simulink model "DynamicModel_Unicycle"  (R2018a)
settings: Solver=ode4  StartTime=0.0  StopTime=10  FixedStep=0.01  RelTol=1e-3
settings Model: Creator=Yuri  LastModifiedBy=Yuri

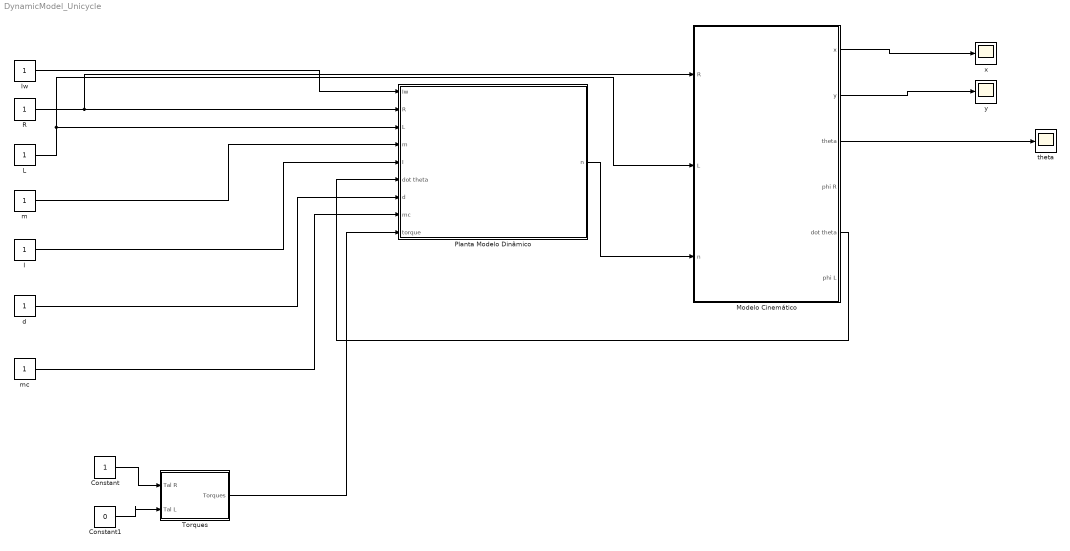
== system DynamicModel_Unicycle ==
  Constant : Constant
  Constant1 : Constant  Value=0
  I : Constant
  Iw : Constant
  L : Constant
  Modelo Cinemático : Subsystem
  Planta Modelo Dinâmico : Subsystem
  R : Constant
  Torques : Subsystem
  d : Constant
  m : Constant
  mc : Constant
  "theta " : Scope
  x : Scope
  y : Scope
  wires:
  R/1 -> Modelo Cinemático/1(R), Planta Modelo Dinâmico/2(R)
  L/1 -> Modelo Cinemático/2(L), Planta Modelo Dinâmico/3(L)
  Iw/1 -> Planta Modelo Dinâmico/1(Iw)
  m/1 -> Planta Modelo Dinâmico/4(m)
  I/1 -> Planta Modelo Dinâmico/5(I)
  d/1 -> Planta Modelo Dinâmico/7(d)
  mc/1 -> Planta Modelo Dinâmico/8(mc)
  Torques/1("Torques ") -> Planta Modelo Dinâmico/9(torque)
  Constant/1 -> Torques/1(Tal R)
  Constant1/1 -> Torques/2(Tal L)
  Modelo Cinemático/3(theta) -> "theta "/1
  Planta Modelo Dinâmico/1(n) -> Modelo Cinemático/3(n)
  Modelo Cinemático/1(x) -> x/1
  Modelo Cinemático/2(y) -> y/1
  Modelo Cinemático/5(dot theta) -> Planta Modelo Dinâmico/6(dot theta)

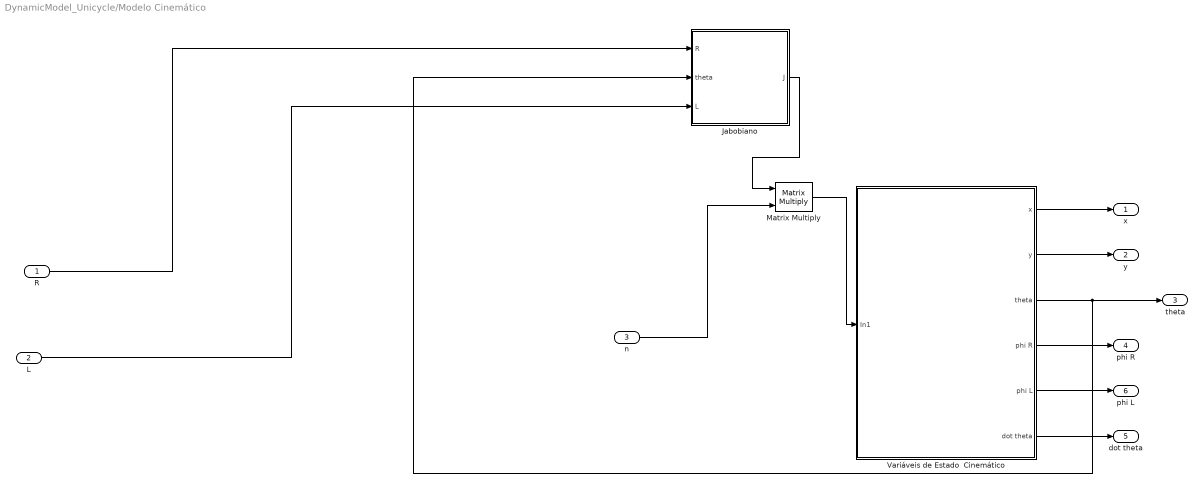
== system DynamicModel_Unicycle/Modelo Cinemático ==
  R : Inport
  L : Inport  Port=2
  n : Inport  Port=3
  "Jabobiano " : Subsystem
  Matrix Multiply : Product  Multiplication=Matrix(*)
  Variáveis de Estado  Cinemático : Subsystem
  x : Outport
  y : Outport  Port=2
  theta : Outport  Port=3
  phi R : Outport  Port=4
  dot theta : Outport  Port=5
  phi L : Outport  Port=6
  wires:
  Matrix Multiply/1 -> Variáveis de Estado  Cinemático/1(In1)
  "Jabobiano "/1(J) -> Matrix Multiply/1
  Variáveis de Estado  Cinemático/5(phi L) -> phi L/1
  Variáveis de Estado  Cinemático/1(x) -> x/1
  Variáveis de Estado  Cinemático/3(theta) -> theta/1, "Jabobiano "/2(theta)
  Variáveis de Estado  Cinemático/6(dot theta) -> dot theta/1
  R/1 -> "Jabobiano "/1(R)
  Variáveis de Estado  Cinemático/4(phi R) -> phi R/1
  Variáveis de Estado  Cinemático/2(y) -> y/1
  L/1 -> "Jabobiano "/3(L)
  n/1 -> Matrix Multiply/2

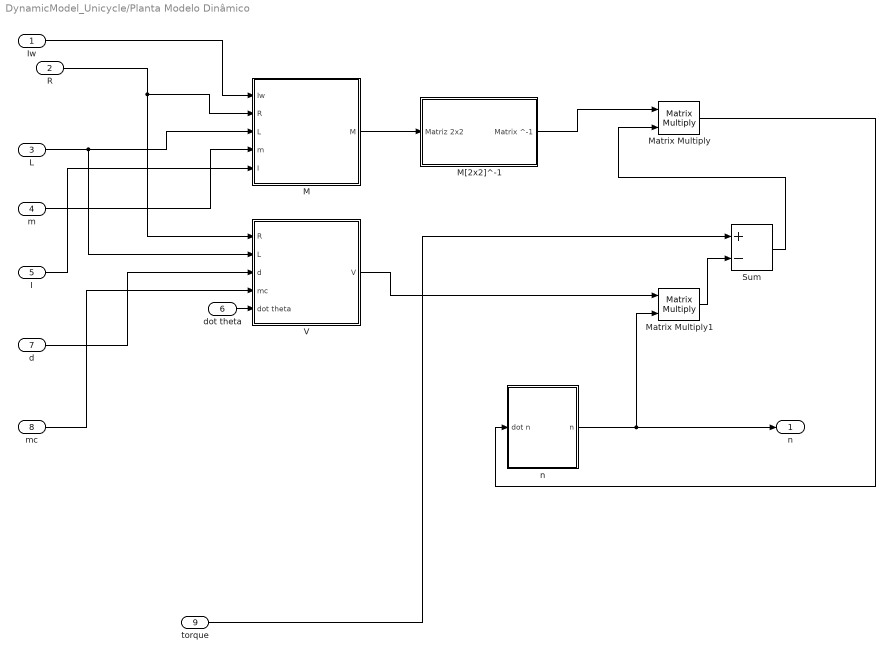
== system DynamicModel_Unicycle/Planta Modelo Dinâmico ==
  Iw : Inport
  R : Inport  Port=2
  L : Inport  Port=3
  m : Inport  Port=4
  I : Inport  Port=5
  dot theta : Inport  Port=6
  d : Inport  Port=7
  mc : Inport  Port=8
  torque : Inport  Port=9
  " n" : Subsystem
  M : Subsystem
  M[2x2]^-1 : Subsystem
  Matrix Multiply : Product  Multiplication=Matrix(*)
  Matrix Multiply1 : Product  Multiplication=Matrix(*)
  Sum : Sum  Inputs=+-
  V : Subsystem
  n : Outport
  wires:
  Matrix Multiply1/1 -> Sum/2
  Sum/1 -> Matrix Multiply/2
  " n"/1("n ") -> n/1, Matrix Multiply1/2
  M[2x2]^-1/1(Matrix ^-1) -> Matrix Multiply/1
  Matrix Multiply/1 -> " n"/1(dot n)
  torque/1 -> Sum/1
  L/1 -> V/2(L), M/3(L)
  mc/1 -> V/4(mc)
  R/1 -> M/2(R), V/1(R)
  dot theta/1 -> V/5(dot theta)
  Iw/1 -> M/1(Iw)
  I/1 -> M/5(I)
  m/1 -> M/4(m)
  d/1 -> V/3(d)
  M/1(M) -> M[2x2]^-1/1("Matriz 2x2 ")
  V/1(V) -> Matrix Multiply1/1

== system DynamicModel_Unicycle/Torques ==
  Tal R : Inport
  Tal L : Inport  Port=2
  Mux : Mux  Inputs=2
  "[2,1]" : Reshape  OutputDimensionality=Customize  OutputDimensions=[2,1]
  "Torques " : Outport
  wires:
  Tal R/1 -> Mux/1
  Tal L/1 -> Mux/2
  Mux/1 -> "[2,1]"/1
  "[2,1]"/1 -> "Torques "/1

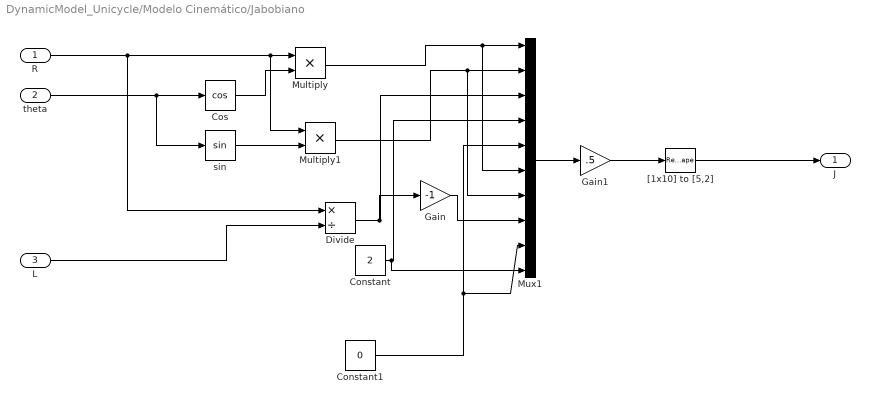
== system DynamicModel_Unicycle/Modelo Cinemático/Jabobiano  ==
  R : Inport
  theta : Inport  Port=2
  L : Inport  Port=3
  Constant : Constant  Value=2
  Constant1 : Constant  Value=0
  Cos : Trigonometry  Operator=cos
  Divide : Product  Inputs=*/
  Gain : Gain  Gain=-1
  Gain1 : Gain  Gain=.5
  Multiply : Product
  Multiply1 : Product
  Mux1 : Mux  Inputs=10
  "[1x10] to [5,2]" : Reshape  OutputDimensionality=Customize  OutputDimensions=[5,2]
  sin : Trigonometry
  J : Outport
  wires:
  R/1 -> Divide/1, Multiply1/1, Multiply/1
  L/1 -> Divide/2
  Mux1/1 -> Gain1/1
  theta/1 -> sin/1, Cos/1
  Cos/1 -> Multiply/2
  Multiply/1 -> Mux1/6, Mux1/1
  sin/1 -> Multiply1/2
  Divide/1 -> Mux1/3, Gain/1
  Constant/1 -> Mux1/10, Mux1/4
  "[1x10] to [5,2]"/1 -> J/1
  Gain1/1 -> "[1x10] to [5,2]"/1
  Multiply1/1 -> Mux1/7, Mux1/2
  Constant1/1 -> Mux1/9, Mux1/5
  Gain/1 -> Mux1/8

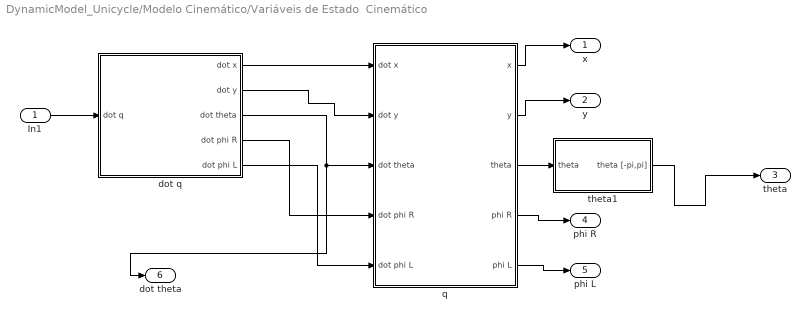
== system DynamicModel_Unicycle/Modelo Cinemático/Variáveis de Estado  Cinemático ==
  In1 : Inport
  " q" : Subsystem
  dot q : Subsystem
  theta1 : Subsystem
  x : Outport
  y : Outport  Port=2
  theta : Outport  Port=3
  phi R : Outport  Port=4
  phi L : Outport  Port=5
  dot theta : Outport  Port=6
  wires:
  dot q/1(dot x) -> " q"/1(dot x)
  dot q/4(dot phi R) -> " q"/4(dot phi R)
  dot q/3(dot theta) -> dot theta/1, " q"/3(dot theta)
  dot q/5(dot phi L) -> " q"/5(dot phi L)
  dot q/2(dot y) -> " q"/2(dot y)
  " q"/5(" phi L") -> phi L/1
  In1/1 -> dot q/1(dot q)
  " q"/4(" phi R") -> phi R/1
  " q"/1(" x") -> x/1
  " q"/2(" y") -> y/1
  " q"/3(" theta") -> theta1/1(theta)
  theta1/1(theta [-pi,pi]) -> theta/1

== system DynamicModel_Unicycle/Planta Modelo Dinâmico/ n ==
  dot n : Inport
  Demux : Demux  Outputs=2
  Integrator : Integrator
  Integrator1 : Integrator
  Mux : Mux  Inputs=2
  "[2,1]" : Reshape  OutputDimensionality=Customize  OutputDimensions=[2,1]
  "n " : Outport
  wires:
  dot n/1 -> Demux/1
  Demux/1 -> Integrator/1
  Demux/2 -> Integrator1/1
  Integrator1/1 -> Mux/2
  Integrator/1 -> Mux/1
  Mux/1 -> "[2,1]"/1
  "[2,1]"/1 -> "n "/1

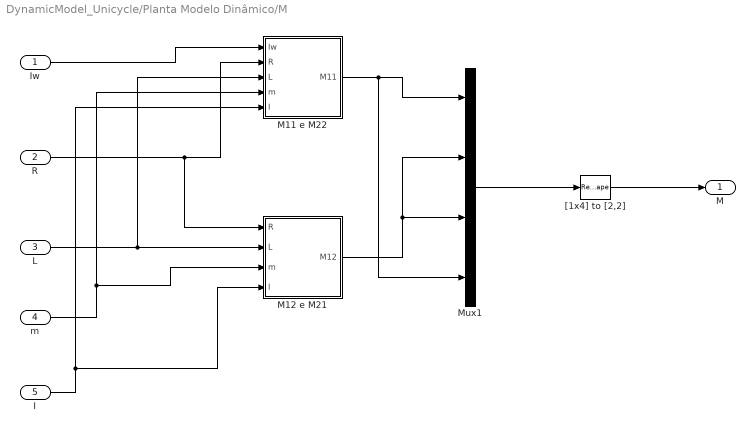
== system DynamicModel_Unicycle/Planta Modelo Dinâmico/M ==
  Iw : Inport
  R : Inport  Port=2
  L : Inport  Port=3
  m : Inport  Port=4
  I : Inport  Port=5
  M11 e M22 : Subsystem
  M12 e M21 : Subsystem
  Mux1 : Mux
  "[1x4] to [2,2]" : Reshape  OutputDimensionality=Customize  OutputDimensions=[2,2]
  M : Outport
  wires:
  Iw/1 -> M11 e M22/1(Iw)
  Mux1/1 -> "[1x4] to [2,2]"/1
  R/1 -> M12 e M21/1(R), M11 e M22/2(R)
  L/1 -> M12 e M21/2(L), M11 e M22/3(L)
  m/1 -> M12 e M21/3("m "), M11 e M22/4("m ")
  I/1 -> M12 e M21/4(I), M11 e M22/5(I)
  M11 e M22/1(M11) -> Mux1/4, Mux1/1
  M12 e M21/1(M12) -> Mux1/3, Mux1/2
  "[1x4] to [2,2]"/1 -> M/1

== system DynamicModel_Unicycle/Planta Modelo Dinâmico/M[2x2]^-1 ==
  "Matriz 2x2 " : Inport
  Demux : Demux
  Gain : Gain  Gain=-1
  Gain1 : Gain  Gain=-1
  Mux : Mux
  Reshape : Reshape  OutputDimensionality=Customize  OutputDimensions=[4,1]
  Reshape1 : Reshape  OutputDimensionality=Customize  OutputDimensions=[2,2]
  Matrix ^-1 : Outport
  wires:
  "Matriz 2x2 "/1 -> Reshape/1
  Demux/1 -> Mux/4
  Demux/4 -> Mux/1
  Demux/2 -> Gain/1
  Gain/1 -> Mux/2
  Demux/3 -> Gain1/1
  Gain1/1 -> Mux/3
  Mux/1 -> Reshape1/1
  Reshape/1 -> Demux/1
  Reshape1/1 -> Matrix ^-1/1

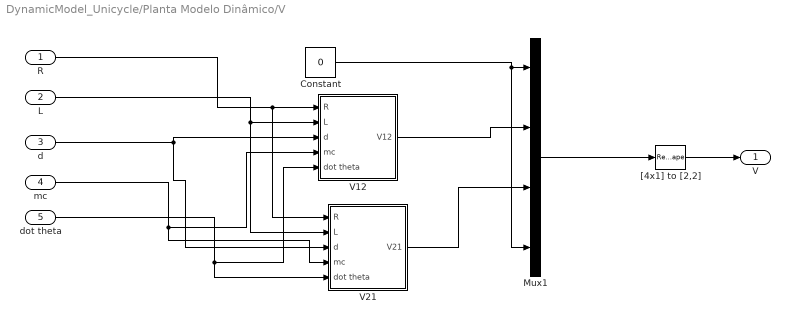
== system DynamicModel_Unicycle/Planta Modelo Dinâmico/V ==
  R : Inport
  L : Inport  Port=2
  d : Inport  Port=3
  mc : Inport  Port=4
  dot theta : Inport  Port=5
  Constant : Constant  Value=0
  Mux1 : Mux
  V12 : Subsystem
  V21 : Subsystem
  "[4x1] to [2,2]" : Reshape  OutputDimensionality=Customize  OutputDimensions=[2,2]
  V : Outport
  wires:
  Constant/1 -> Mux1/4, Mux1/1
  V12/1("V12 ") -> Mux1/2
  V21/1("V21 ") -> Mux1/3
  R/1 -> V21/1(R), V12/1(R)
  L/1 -> V21/2(L), V12/2(L)
  d/1 -> V21/3(d), V12/3(d)
  dot theta/1 -> V21/5(dot theta), V12/5(dot theta)
  mc/1 -> V21/4(mc), V12/4(mc)
  Mux1/1 -> "[4x1] to [2,2]"/1
  "[4x1] to [2,2]"/1 -> V/1

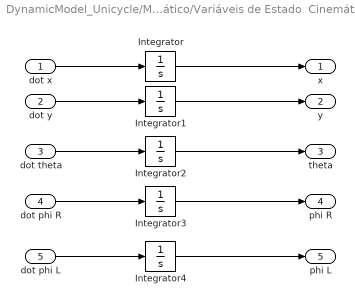
== system DynamicModel_Unicycle/Modelo Cinemático/Variáveis de Estado  Cinemático/ q ==
  dot x : Inport
  dot y : Inport  Port=2
  dot theta : Inport  Port=3
  dot phi R : Inport  Port=4
  dot phi L : Inport  Port=5
  Integrator{,1..4} (5 alike) : Integrator
  " x" : Outport
  " y" : Outport  Port=2
  " theta" : Outport  Port=3
  " phi R" : Outport  Port=4
  " phi L" : Outport  Port=5
  wires:
  dot x/1 -> Integrator/1
  Integrator/1 -> " x"/1
  dot y/1 -> Integrator1/1
  Integrator1/1 -> " y"/1
  dot theta/1 -> Integrator2/1
  Integrator2/1 -> " theta"/1
  dot phi R/1 -> Integrator3/1
  Integrator3/1 -> " phi R"/1
  dot phi L/1 -> Integrator4/1
  Integrator4/1 -> " phi L"/1

== system DynamicModel_Unicycle/Modelo Cinemático/Variáveis de Estado  Cinemático/dot q ==
  dot q : Inport
  Demux : Demux  Outputs=5
  dot x : Outport
  dot y : Outport  Port=2
  dot theta : Outport  Port=3
  dot phi R : Outport  Port=4
  dot phi L : Outport  Port=5
  wires:
  Demux/2 -> dot y/1
  dot q/1 -> Demux/1
  Demux/1 -> dot x/1
  Demux/3 -> dot theta/1
  Demux/4 -> dot phi R/1
  Demux/5 -> dot phi L/1

== system DynamicModel_Unicycle/Modelo Cinemático/Variáveis de Estado  Cinemático/theta1 ==
  theta : Inport
  Atan : Trigonometry  Operator=atan
  Cos : Trigonometry  Operator=cos
  Divide : Product  Inputs=*/
  Sin : Trigonometry
  theta [-pi,pi] : Outport
  wires:
  theta/1 -> Cos/1, Sin/1
  Cos/1 -> Divide/2
  Sin/1 -> Divide/1
  Divide/1 -> Atan/1
  Atan/1 -> theta [-pi,pi]/1

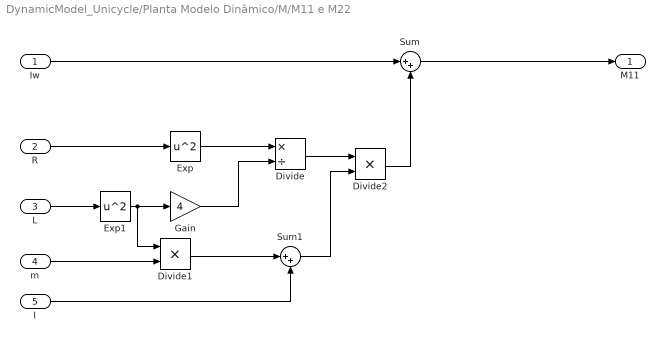
== system DynamicModel_Unicycle/Planta Modelo Dinâmico/M/M11 e M22 ==
  Iw : Inport
  R : Inport  Port=2
  L : Inport  Port=3
  "m " : Inport  Port=4
  I : Inport  Port=5
  Divide : Product  Inputs=*/
  Divide1 : Product  Inputs=**
  Divide2 : Product  Inputs=**
  Exp : Math  Operator=square  SaturateOnIntegerOverflow=on
  Exp1 : Math  Operator=square  SaturateOnIntegerOverflow=on
  Gain : Gain  Gain=4
  Sum : Sum  Inputs=|++
  Sum1 : Sum  Inputs=|++
  M11 : Outport
  wires:
  Iw/1 -> Sum/1
  Sum/1 -> M11/1
  R/1 -> Exp/1
  Exp/1 -> Divide/1
  L/1 -> Exp1/1
  Exp1/1 -> Divide1/1, Gain/1
  Gain/1 -> Divide/2
  "m "/1 -> Divide1/2
  Divide1/1 -> Sum1/1
  I/1 -> Sum1/2
  Divide/1 -> Divide2/1
  Sum1/1 -> Divide2/2
  Divide2/1 -> Sum/2

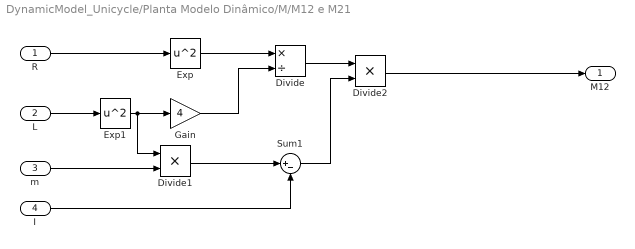
== system DynamicModel_Unicycle/Planta Modelo Dinâmico/M/M12 e M21 ==
  R : Inport
  L : Inport  Port=2
  "m " : Inport  Port=3
  I : Inport  Port=4
  Divide : Product  Inputs=*/
  Divide1 : Product  Inputs=**
  Divide2 : Product  Inputs=**
  Exp : Math  Operator=square  SaturateOnIntegerOverflow=on
  Exp1 : Math  Operator=square  SaturateOnIntegerOverflow=on
  Gain : Gain  Gain=4
  Sum1 : Sum  Inputs=|+-
  M12 : Outport
  wires:
  Divide2/1 -> M12/1
  R/1 -> Exp/1
  Exp/1 -> Divide/1
  L/1 -> Exp1/1
  Exp1/1 -> Divide1/1, Gain/1
  Gain/1 -> Divide/2
  "m "/1 -> Divide1/2
  Divide1/1 -> Sum1/1
  I/1 -> Sum1/2
  Divide/1 -> Divide2/1
  Sum1/1 -> Divide2/2

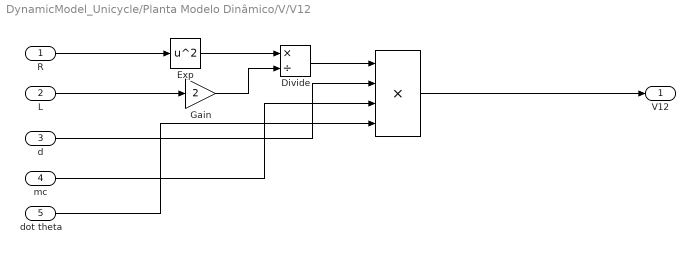
== system DynamicModel_Unicycle/Planta Modelo Dinâmico/V/V12 ==
  R : Inport
  L : Inport  Port=2
  d : Inport  Port=3
  mc : Inport  Port=4
  dot theta : Inport  Port=5
  " " : Product  Inputs=****
  Divide : Product  Inputs=*/
  Exp : Math  Operator=square  SaturateOnIntegerOverflow=on
  Gain : Gain  Gain=2
  "V12 " : Outport
  wires:
  Exp/1 -> Divide/1
  L/1 -> Gain/1
  Gain/1 -> Divide/2
  R/1 -> Exp/1
  Divide/1 -> " "/1
  d/1 -> " "/2
  mc/1 -> " "/3
  dot theta/1 -> " "/4
  " "/1 -> "V12 "/1

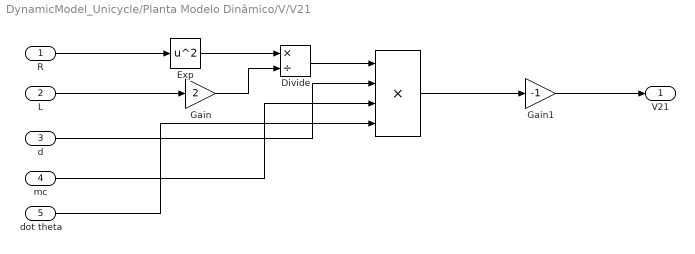
== system DynamicModel_Unicycle/Planta Modelo Dinâmico/V/V21 ==
  R : Inport
  L : Inport  Port=2
  d : Inport  Port=3
  mc : Inport  Port=4
  dot theta : Inport  Port=5
  " " : Product  Inputs=****
  Divide : Product  Inputs=*/
  Exp : Math  Operator=square  SaturateOnIntegerOverflow=on
  Gain : Gain  Gain=2
  Gain1 : Gain  Gain=-1
  "V21 " : Outport
  wires:
  Exp/1 -> Divide/1
  L/1 -> Gain/1
  Gain/1 -> Divide/2
  R/1 -> Exp/1
  Divide/1 -> " "/1
  d/1 -> " "/2
  mc/1 -> " "/3
  dot theta/1 -> " "/4
  " "/1 -> Gain1/1
  Gain1/1 -> "V21 "/1
